simulink model "motori"  (R2020b)
settings: Solver=VariableStepAuto  StartTime=0.0  StopTime=10.0  RelTol=1e-3
settings Model: Creator=fiori  LastModifiedBy=fiori

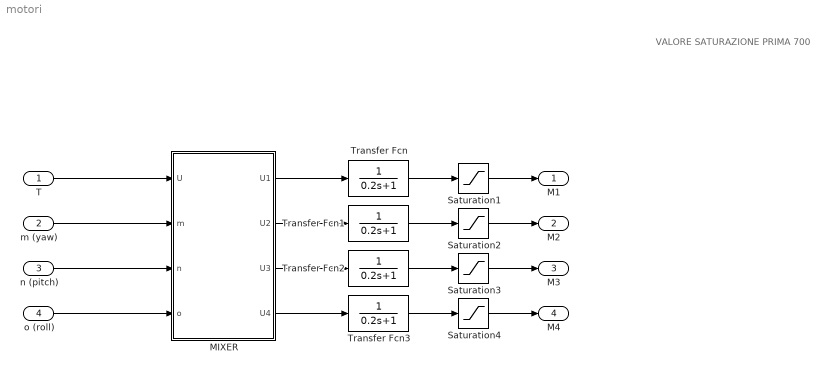
== system motori ==
  note: VALORE SATURAZIONE PRIMA 700
  T : Inport
  m (yaw) : Inport  Port=2
  n (pitch) : Inport  Port=3
  o (roll) : Inport  Port=4
  MIXER : MATLAB Function  TreatAsAtomicUnit=on
  Saturation{1..4} (4 alike) : Saturate  UpperLimit=850  LowerLimit=0
  Transfer Fcn{,1..3} (4 alike) : TransferFcn  Denominator=[0.2 1]
  M1 : Outport
  M2 : Outport  Port=2
  M3 : Outport  Port=3
  M4 : Outport  Port=4
  wires:
  m (yaw)/1 -> MIXER/2(m)
  Saturation1/1 -> M1/1
  Transfer Fcn/1 -> Saturation1/1
  Transfer Fcn2/1 -> Saturation3/1
  n (pitch)/1 -> MIXER/3(n)
  T/1 -> MIXER/1(U)
  Transfer Fcn1/1 -> Saturation2/1
  MIXER/2(U2) -> Transfer Fcn1/1
  MIXER/3(U3) -> Transfer Fcn2/1
  o (roll)/1 -> MIXER/4(o)
  Transfer Fcn3/1 -> Saturation4/1
  MIXER/4(U4) -> Transfer Fcn3/1
  Saturation3/1 -> M3/1
  Saturation2/1 -> M2/1
  MIXER/1(U1) -> Transfer Fcn/1
  Saturation4/1 -> M4/1

== matlab function motori/MIXER ==
  data: U input; U1 output; m input; n input; o input; U2 output; U3 output; U4 output
function [U1,U2,U3,U4] = motormix(U,m,n,o)
U24=(m+1)*U;
U13=(1-m)*U;

U1=(n+1)*U13;
U3=(1-n)*U13;

U2=(o+1)*U24;
U4=(1-o)*U24;
